simulink model "top_model"  (R2017a)
settings: Solver=ode23t  StartTime=0.0  StopTime=100  FixedStep=0.005  MaxStep=0.05  RelTol=1e-8  EnableMultiTasking=on
InitFcn:
  | load('DrivenData.mat');
  | load('vehicleParameters.mat');
undefined symbols (not defined in the file): B, C, CA, Cd, Cl, cogHeight, D, E, F, frontArea, frontBrakeBias, mass, maxBrakingTorque, maxPower, maxTorque, P, R, rearWeightDist, trackWidth, wheelBase
(part 2 of 2)

== system top_model/Vehicle/Wheels/Tire Forces/Pacejka Function Slip Angle ==
  x : Inport
  "B " : Inport  Port=2
  C : Inport  Port=3
  D : Inport  Port=4
  E : Inport  Port=5
  Bx : Product
  Bx - E(Bx - arctan(Bx) : Sum  Inputs=+-
  Bx - arctan(Bx) : Sum  Inputs=+-
  C(arctan(Bx - E(Bx - arctan(Bx)))) : Product
  D[sin(C(arctan(Bx - E(Bx - arctan(Bx)))))] : Product
  E(Bx - arctan(Bx) : Product
  arctan(Bx - E(Bx - arctan(Bx))) : Trigonometry  Operator=atan
  arctan(Bx) : Trigonometry  Operator=atan
  sin(C(arctan(Bx - E(Bx - arctan(Bx))))) : Trigonometry
  y : Outport
  wires:
  D/1 -> D[sin(C(arctan(Bx - E(Bx - arctan(Bx)))))]/2
  x/1 -> Bx/1
  Bx - E(Bx - arctan(Bx)/1 -> arctan(Bx - E(Bx - arctan(Bx)))/1
  C(arctan(Bx - E(Bx - arctan(Bx))))/1 -> sin(C(arctan(Bx - E(Bx - arctan(Bx)))))/1
  D[sin(C(arctan(Bx - E(Bx - arctan(Bx)))))]/1 -> y/1
  Bx - arctan(Bx)/1 -> E(Bx - arctan(Bx)/1
  E(Bx - arctan(Bx)/1 -> Bx - E(Bx - arctan(Bx)/2
  arctan(Bx - E(Bx - arctan(Bx)))/1 -> C(arctan(Bx - E(Bx - arctan(Bx))))/1
  arctan(Bx)/1 -> Bx - arctan(Bx)/2
  "B "/1 -> Bx/2
  E/1 -> E(Bx - arctan(Bx)/2
  sin(C(arctan(Bx - E(Bx - arctan(Bx)))))/1 -> D[sin(C(arctan(Bx - E(Bx - arctan(Bx)))))]/1
  C/1 -> C(arctan(Bx - E(Bx - arctan(Bx))))/2
  Bx/1 -> Bx - E(Bx - arctan(Bx)/1, Bx - arctan(Bx)/1, arctan(Bx)/1

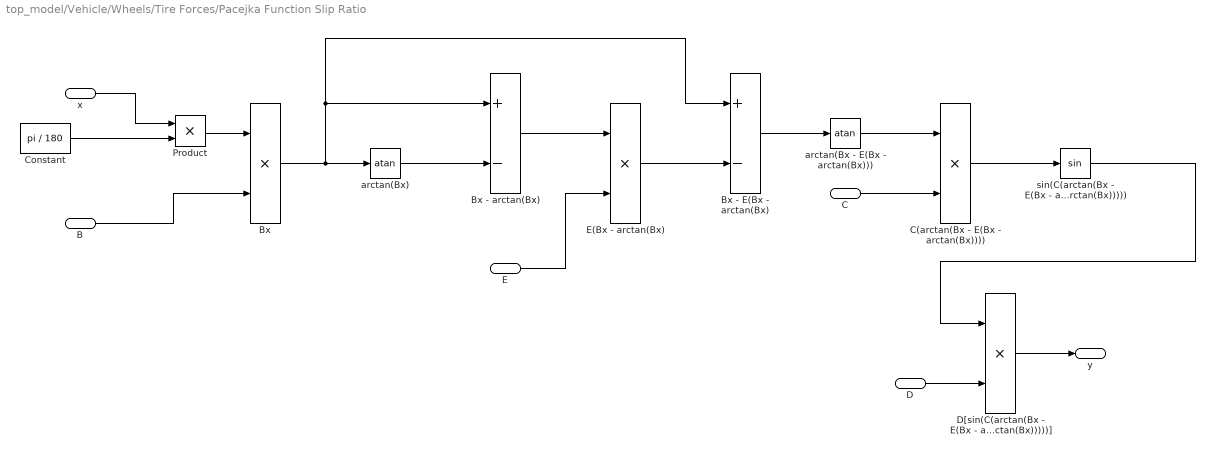
== system top_model/Vehicle/Wheels/Tire Forces/Pacejka Function Slip Ratio ==
  x : Inport
  "B " : Inport  Port=2
  C : Inport  Port=3
  D : Inport  Port=4
  E : Inport  Port=5
  Bx : Product
  Bx - E(Bx - arctan(Bx) : Sum  Inputs=+-
  Bx - arctan(Bx) : Sum  Inputs=+-
  C(arctan(Bx - E(Bx - arctan(Bx)))) : Product
  Constant : Constant  Value=pi / 180
  D[sin(C(arctan(Bx - E(Bx - arctan(Bx)))))] : Product
  E(Bx - arctan(Bx) : Product
  Product : Product
  arctan(Bx - E(Bx - arctan(Bx))) : Trigonometry  Operator=atan
  arctan(Bx) : Trigonometry  Operator=atan
  sin(C(arctan(Bx - E(Bx - arctan(Bx))))) : Trigonometry
  y : Outport
  wires:
  D/1 -> D[sin(C(arctan(Bx - E(Bx - arctan(Bx)))))]/2
  Bx - E(Bx - arctan(Bx)/1 -> arctan(Bx - E(Bx - arctan(Bx)))/1
  C(arctan(Bx - E(Bx - arctan(Bx))))/1 -> sin(C(arctan(Bx - E(Bx - arctan(Bx)))))/1
  D[sin(C(arctan(Bx - E(Bx - arctan(Bx)))))]/1 -> y/1
  Bx - arctan(Bx)/1 -> E(Bx - arctan(Bx)/1
  E(Bx - arctan(Bx)/1 -> Bx - E(Bx - arctan(Bx)/2
  arctan(Bx - E(Bx - arctan(Bx)))/1 -> C(arctan(Bx - E(Bx - arctan(Bx))))/1
  arctan(Bx)/1 -> Bx - arctan(Bx)/2
  E/1 -> E(Bx - arctan(Bx)/2
  sin(C(arctan(Bx - E(Bx - arctan(Bx)))))/1 -> D[sin(C(arctan(Bx - E(Bx - arctan(Bx)))))]/1
  C/1 -> C(arctan(Bx - E(Bx - arctan(Bx))))/2
  Bx/1 -> Bx - E(Bx - arctan(Bx)/1, Bx - arctan(Bx)/1, arctan(Bx)/1
  Constant/1 -> Product/2
  Product/1 -> Bx/1
  x/1 -> Product/1
  "B "/1 -> Bx/2

== system top_model/Vehicle/Wheels/Tire Forces/Slip Ratio Multiplier ==
  maxFY : Inport
  Slip Ratio : Inport  Port=2
  R : Inport  Port=3
  Abs : Abs
  Constant : Constant
  Constant1 : Constant  Value=0
  Product : Product
  Product1 : Product
  Subtract : Sum  Inputs=+-
  lower bound : MinMax  Function=max  Inputs=2
  FY : Outport
  wires:
  Abs/1 -> Product/1
  Product/1 -> Subtract/2
  Constant/1 -> Subtract/1
  maxFY/1 -> Product1/1
  Product1/1 -> FY/1
  R/1 -> Product/2
  Slip Ratio/1 -> Abs/1
  Subtract/1 -> lower bound/1
  Constant1/1 -> lower bound/2
  lower bound/1 -> Product1/2
